simulink model "SF013A_PullCmpActv"  (R2013b)
settings: Solver=FixedStepDiscrete  SolverMode=SingleTasking  StartTime=0.0  StopTime=1  FixedStep=0.002  RelTol=1e-3
values from neighbouring files (symbols this model uses):
  ARCHGLBPRM_100MILLISEC_SEC_F32 = DataDict.Constant    [SF013A_PullCmpActv_DataDict.m]
  ARCHGLBPRM_2MILLISEC_SEC_F32 = DataDict.Constant    [SF013A_PullCmpActv_DataDict.m]
  ARCHGLBPRM_FLOATZEROTHD_ULS_F32 = DataDict.Constant    [SF013A_PullCmpActv_DataDict.m]
  INTGTRSCARSHOTERM_ULS_F32 = DataDict.Constant    [SF013A_PullCmpActv_DataDict.m]
  LONGTERMINTGTRSCAR_ULS_F32 = DataDict.Constant    [SF013A_PullCmpActv_DataDict.m]
  MICROSECTOSEC_ULS_F32 = DataDict.Constant    [SF013A_PullCmpActv_DataDict.m]
  MINSTOSEC_SECPERMINS_F32 = DataDict.Constant    [SF013A_PullCmpActv_DataDict.m]
  PullCmpActvCmpLrnTiDecShoTerm = DataDict.Calibration    [SF013A_PullCmpActv_DataDict.m]
  PullCmpActvCmpLrnTiIncShoTerm = DataDict.Calibration    [SF013A_PullCmpActv_DataDict.m]
  PullCmpActvCmpLrnTiLongTerm = DataDict.Calibration    [SF013A_PullCmpActv_DataDict.m]
  PullCmpActvCmpShoTermRstHwAgThd = DataDict.Calibration    [SF013A_PullCmpActv_DataDict.m]
  PullCmpActvCmpShoTermRstHwTqThd = DataDict.Calibration    [SF013A_PullCmpActv_DataDict.m]
  PullCmpActvCmpShoTermRstLatAThd = DataDict.Calibration    [SF013A_PullCmpActv_DataDict.m]
  PullCmpActvCmpShoTermRstYawRateThd = DataDict.Calibration    [SF013A_PullCmpActv_DataDict.m]
  PullCmpActvEna = DataDict.Calibration    [SF013A_PullCmpActv_DataDict.m]
  PullCmpActvLongTermLim = DataDict.Calibration    [SF013A_PullCmpActv_DataDict.m]
  PullCmpActvLrngEnaAgConfMinMgn = DataDict.Calibration    [SF013A_PullCmpActv_DataDict.m]
  PullCmpActvLrngEnaHwAgMaxMgn = DataDict.Calibration    [SF013A_PullCmpActv_DataDict.m]
  PullCmpActvLrngEnaHwTqMaxMgn = DataDict.Calibration    [SF013A_PullCmpActv_DataDict.m]
  PullCmpActvLrngEnaHwVelMaxMgn = DataDict.Calibration    [SF013A_PullCmpActv_DataDict.m]
  PullCmpActvLrngEnaLatAMaxMgn = DataDict.Calibration    [SF013A_PullCmpActv_DataDict.m]
  PullCmpActvLrngEnaTiThd = DataDict.Calibration    [SF013A_PullCmpActv_DataDict.m]
  PullCmpActvLrngEnaVehSpdMaxMgn = DataDict.Calibration    [SF013A_PullCmpActv_DataDict.m]
  PullCmpActvLrngEnaVehSpdMinMgn = DataDict.Calibration    [SF013A_PullCmpActv_DataDict.m]
  PullCmpActvLrngEnaVehSpdRateMaxMgn = DataDict.Calibration    [SF013A_PullCmpActv_DataDict.m]
  PullCmpActvLrngEnaYawRateMaxMgn = DataDict.Calibration    [SF013A_PullCmpActv_DataDict.m]
  PullCmpActvOpstSignTiShoTerm = DataDict.Calibration    [SF013A_PullCmpActv_DataDict.m]
  PullCmpActvOutpMaxRate = DataDict.Calibration    [SF013A_PullCmpActv_DataDict.m]
  PullCmpActvPullCmpShoTermLim = DataDict.Calibration    [SF013A_PullCmpActv_DataDict.m]
  PullCmpActvPullCmpTotLim = DataDict.Calibration    [SF013A_PullCmpActv_DataDict.m]
  PullCmpActvPullErrLimLongTerm = DataDict.Calibration    [SF013A_PullCmpActv_DataDict.m]
  PullCmpActvPullErrMgnThd = DataDict.Calibration    [SF013A_PullCmpActv_DataDict.m]
  PullCmpActvPullErrShoTermLim = DataDict.Calibration    [SF013A_PullCmpActv_DataDict.m]
  PullCmpActvShoTermRampTi = DataDict.Calibration    [SF013A_PullCmpActv_DataDict.m]
  SysGlbPrmSysTqRat = DataDict.ImprtdCal    [SF013A_PullCmpActv_DataDict.m]
libraries: NxtrAbslt x9, Fil x8, NxtrLim x6, FixdToFloat x3, NxtrSign x3, NxtrMin x3, NxtrNvM x2, NxtrMax x2, simulink x1, FloatToFixd x1, LnrIntrpn x1
(part 1 of 3)
settings Model: Creator=DZVCQL  LastModifiedBy=XZB1DB
settings SolverCC: AutoInsertRateTranBlk=on  InsertRTBMode=Always
settings DataIOCC: LimitDataPoints=off  SaveFormat=Structure  ReturnWorkspaceOutputs=on
settings OptimizationCC: BlockReduction=off  InlineParams=on  ZeroExternalMemoryAtStartup=off  ZeroInternalMemoryAtStartup=off  OptimizeModelRefInitCode=on  LifeSpan=1
settings DebuggingCC: SignalInfNanChecking=error  SignalRangeChecking=warning  ReadBeforeWriteMsg=DisableAll  WriteAfterWriteMsg=DisableAll  WriteAfterReadMsg=DisableAll  UnderspecifiedInitializationDetection=Simplified  SolverPrmCheckMsg=error  InheritedTsInSrcMsg=error  DiscreteInheritContinuousMsg=error  SingleTaskRateTransMsg=error  TasksWithSamePriorityMsg=error  SigSpecEnsureSampleTimeMsg=error  CheckMatrixSingularityMsg=error  ParameterUnderflowMsg=error  ParameterPrecisionLossMsg=error  ParameterTunabilityLossMsg=error  FixptConstUnderflowMsg=warning  FixptConstOverflowMsg=warning  VectorMatrixConversionMsg=error  SignalLabelMismatchMsg=error  UnconnectedInputMsg=error  UnconnectedOutputMsg=error  UnconnectedLineMsg=error  SFcnCompatibilityMsg=error  UniqueDataStoreMsg=warning  BusObjectLabelMismatch=error  RootOutportRequireBusObject=error  AssertControl=DisableAll  ModelReferenceIOMsg=error  ModelReferenceVersionMismatchMessage=warning  ModelReferenceIOMismatchMessage=error  ModelReferenceCSMismatchMessage=warning  ModelReferenceDataLoggingMessage=error  StateNameClashWarn=warning  StrictBusMsg=ErrorOnBusTreatedAsVector  NonBusSignalsTreatedAsBus=error  SFUnexpectedBacktrackingDiag=error  SFInvalidInputDataAccessInChartInitDiag=error  SFNoUnconditionalDefaultTransitionDiag=error  SFTransitionOutsideNaturalParentDiag=error  SFUnconditionalTransitionShadowingDiag=error  SFUndirectedBroadcastEventsDiag=error
settings ModelReferenceCC: ModelReferenceNumInstancesAllowed=Single
settings RTWCC: SystemTargetFile=autosar.tlc  GenCodeOnly=on  TemplateMakefile=ert_default_tmf  Description=AUTOSAR  GenerateReport=on  ProcessScript=autosar_make_rtw_hook  LaunchReport=on
settings CodeAppCC: GenerateComments=off  IgnoreCustomStorageClasses=off  CustomSymbolStrType=$N$R$M  CustomSymbolStrBlkIO=$N$M  SimulinkBlockComments=off
settings STFCustomTargetCC: ParMdlRefBuildCompliant=on  CompOptLevelCompliant=on  IncludeMdlTerminateFcn=off  CombineOutputUpdateFcns=on  SuppressErrorStatus=on  ERTFirstTimeCompliant=on  ERTCustomFileBanners=on  SupportNonFinite=off  SupportComplex=off  SupportContinuousTime=off  SupportNonInlinedSFcns=off  MATLABClassNameForMDSCustomization=Simulink.SoftwareTarget.ERTCustomization  AutosarCompliant=on  GRTInterface=off  SystemTargetFile=autosar.tlc
settings ERTTargetCC: CodeReplacementLibrary=ANSI_C  ConcurrentExecutionCompliant=off  IncludeMdlTerminateFcn=off  SuppressErrorStatus=on  SupportNonFinite=off  SupportComplex=off  ModelStepFunctionPrototypeControlCompliant=off  CPPClassGenCompliant=off  AutosarCompliant=on  InlinedParameterPlacement=NonHierarchical  ERTCustomFileTemplate=example_file_process.tlc  EnableUserReplacementTypes=on

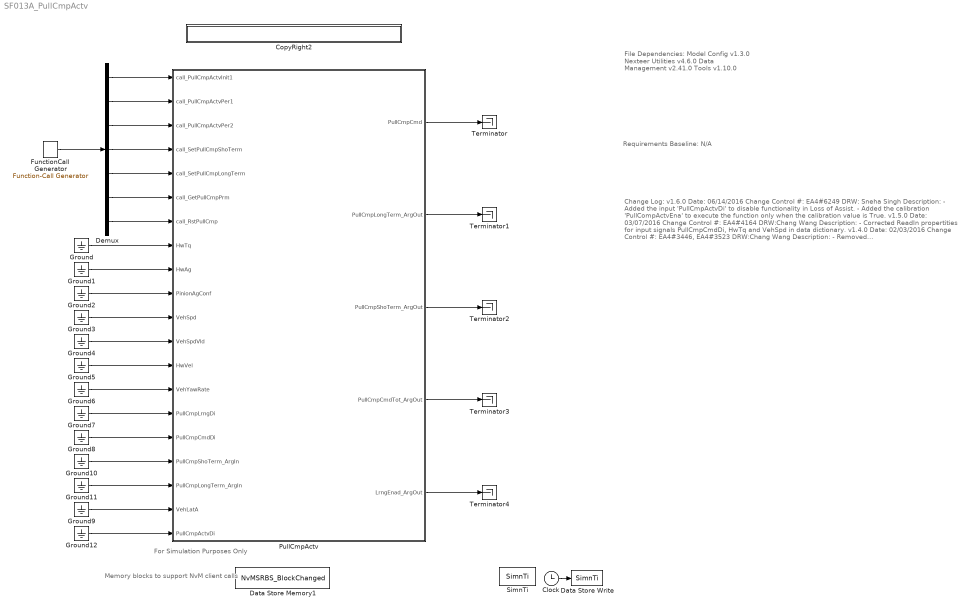
== system SF013A_PullCmpActv ==
  note: Memory blocks to support NvM client calls
  note: For Simulation Purposes Only
  note: File Dependencies:
      |
      | Model Config v1.3.0
      | Nexteer Utilities v4.6.0
      | Data Management v2.41.0
      | Tools v1.10.0
  note: Requirements Baseline: N/A
  note: Change Log:
      |
      | v1.6.0
      | Date: 06/14/2016
      | Change Control #: EA4#6249
      | DRW: Sneha Singh
      | Description:
      | - Added the input 'PullCmpActvDi' to disable functionality in Loss of Assist.
      | - Added the calibration 'PullCompActvEna' to execute the function only when the calibration value is True.
      |
      | v1.5.0
      | Date: 03/07/2016
      | Change Control #: EA4#4164
      | DRW:Chang Wang
      | Description:
      | - Corrected ReadIn propertities for input signals PullCmpCmdDi, HwTq and VehSpd in data dictionary.
      |
      |
      | v1.4.0
      | Date: 02/03/2016
      | Change Control #: EA4#3446, EA4#3523
      | DRW:Chang Wang
      | Description:
      | - Removed PullCmpActvCmpShoTermRstYawRate in the data dictionary as duplicated calibration.
      | - Added VehLatA as the new input to the function for the new functionality, enabling  learning and reset short term learning based on lateral acceleration.
      | - Changed min and max value for PIM PullCmpCmdTot.
      | - Enabled StateMustResolveToSignalObject for IntgtrGainIncShoTerm and IntgtrGainDecShoTerm.
      |
      |
      | v1.3.0
      | Date: 10/15/2015
      | Change Control #: EA4#1967
      | DRW: Price Lefler
      | Description:
      | - Fixed DocUnits for RefTiEnaLrng,  RefTiOpstSign and PullCmpActvOpstSignTiShoTerm.
      | - Fixed design error in the calculation of the short term increasing and decreasing integral gains.
      |
      |
      | v1.2.0
      | Date: 10/2/2015
      | Change Control #: EA4#1009
      | DRW: Price Lefler
      | Description:
      | - Removed GetErrorStatus as a client call in the data dictionary.
      |
      | v1.1.0
      | Date: 9/28/2015
      | Change Control #: EA4#1009
      | DRW: Price Lefler
      | Description:
      | - Timer function usage fixed.
      | - ReadIn and WrittenIn properties fixed for the IRV RampDwnStepSize.
      | - Not equal to comparisons for floating point numbers removed and replaced with a difference and a comparison to ARCHGLBPRM_FLOATZEROTHD_ULS_F32
      | - Removed check of GetErrorStatus for PullCmpLongTerm in the model.
      | - Removed the link to undesired requirement.
      |
      | v1.0.0
      | Date:
      | Change Control #: EA4#1009
      | DRW: Chang Wang
      | Description:
      | - Initial Release
      | - Created from EA3 v003
      | - Level 1 model
  Clock : Clock
  CopyRight2 : Subsystem  Description=|  mask(Copyright Information){none=on}
      | Copyright info block.                                               
      |                                                                     
      | Place copyright information at the top of every subsystem in design.
      mask prompts: none "No parameters"
      mask help: Place copyright information at the top of every subsystem in design.
      mask Display:
      | NxtrConf = 'Nexteer Confidential';
      | 
      | sys = bdroot; %handle for the current model ("system")
      | first = get_param(sys,'Created');
      | if(isempty(first))
      |     first = datestr(now,'yyyy');
      | else
      |     first = first(end-3:end);  %year is last four digits
      | end
      | 
      | last = get_param(sys,'LastModifiedDate');
      | if isempty(last)
      |     last = datestr(now,'yyyy');
      | else
      |     last = last(end-3:end);
      | end
      | 
      | if strcmp(first,last)
      |     fprintf('%s -- Copyright %s Nexteer',NxtrConf,first)
      | else
      |     fprintf('%s -- %s%s- %s Nexteer',NxtrConf,char(169),first,last)
      | end
  Data Store Memory1 : DataStoreMemory  DataStoreName=NvMSRBS_BlockChanged  ReadBeforeWriteMsg=warning  WriteAfterWriteMsg=warning  WriteAfterReadMsg=warning
  Data Store Write : DataStoreWrite  DataStoreName=SimnTi
  Demux : Demux  Outputs=7
  FunctionCall Generator : simulink/Ports & Subsystems/Function-Call Generator  sample_time=0.002  numberOfIterations=1
  Ground{,1..12} (13 alike) : Ground
  PullCmpActv : Subsystem
  SimnTi : DataStoreMemory  DataStoreName=SimnTi
  Terminator{,1..4} (5 alike) : Terminator
  wires:
  Clock/1 -> Data Store Write/1
  Demux/1 -> PullCmpActv/1(call_PullCmpActvInit1)
  Demux/2 -> PullCmpActv/2(call_PullCmpActvPer1)
  FunctionCall Generator/1 -> Demux/1
  Demux/3 -> PullCmpActv/3(call_PullCmpActvPer2)
  Demux/4 -> PullCmpActv/4(call_SetPullCmpShoTerm)
  Demux/5 -> PullCmpActv/5(call_SetPullCmpLongTerm)
  Demux/6 -> PullCmpActv/6(call_GetPullCmpPrm)
  Ground/1 -> PullCmpActv/8(HwTq)
  Ground1/1 -> PullCmpActv/9(HwAg)
  Ground2/1 -> PullCmpActv/10(PinionAgConf)
  Ground3/1 -> PullCmpActv/11(VehSpd)
  Ground4/1 -> PullCmpActv/12(VehSpdVld)
  Ground5/1 -> PullCmpActv/13(HwVel)
  Ground6/1 -> PullCmpActv/14(VehYawRate)
  Ground7/1 -> PullCmpActv/15(PullCmpLrngDi)
  Ground8/1 -> PullCmpActv/16(PullCmpCmdDi)
  Ground10/1 -> PullCmpActv/17(PullCmpShoTerm_ArgIn)
  Ground11/1 -> PullCmpActv/18(PullCmpLongTerm_ArgIn)
  PullCmpActv/1(PullCmpCmd) -> Terminator/1
  PullCmpActv/2(PullCmpLongTerm_ArgOut) -> Terminator1/1
  PullCmpActv/3(PullCmpShoTerm_ArgOut) -> Terminator2/1
  PullCmpActv/4(PullCmpCmdTot_ArgOut) -> Terminator3/1
  PullCmpActv/5(LrngEnad_ArgOut) -> Terminator4/1
  Demux/7 -> PullCmpActv/7(call_RstPullCmp)
  Ground9/1 -> PullCmpActv/19(VehLatA)
  Ground12/1 -> PullCmpActv/20(PullCmpActvDi)

== system SF013A_PullCmpActv/CopyRight2 ==

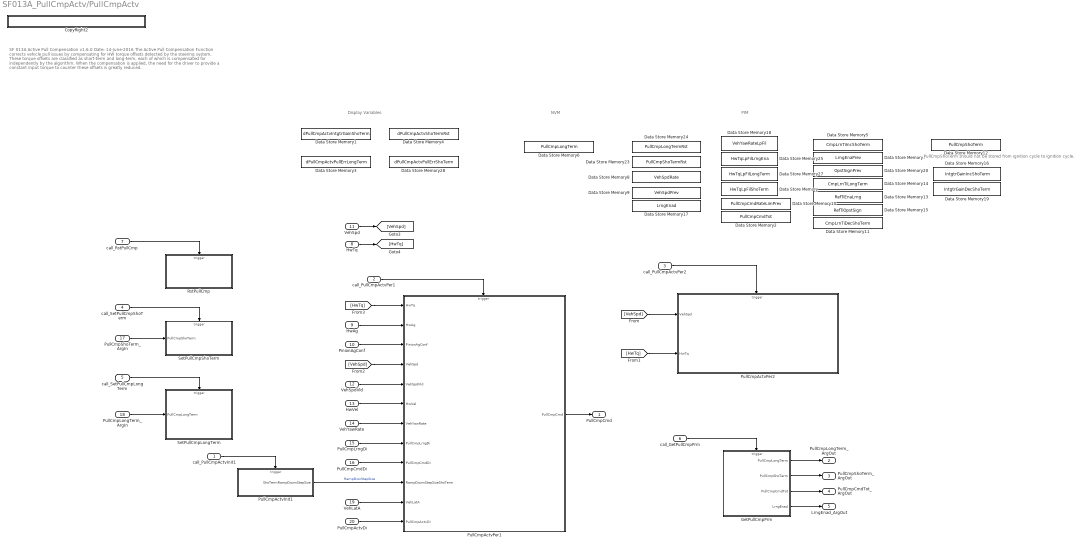
== system SF013A_PullCmpActv/PullCmpActv ==
  note: PullCmpShoTerm should not be stored from ignition cycle to ignition cycle.
  note: Display Variables
  note: SF 013A  Active Pull Compensation
      | v1.6.0      Date: 14-June-2016
      |
      | The Active Pull Compensation Function corrects vehicle pull issues by compensating for HW torque offsets detected by the steering system.
      | These torque offsets are classified as short-term and long-term, each of which is compensated for independently by the algorithm.  When
      | the compensation is applied, the need for the driver to provide a constant input torque to counter these offsets is greatly reduced.
  note: NVM
  note: PIM
  call_PullCmpActvInit1 : Inport
  call_PullCmpActvPer1 : Inport  Port=2
  call_PullCmpActvPer2 : Inport  Port=3
  call_SetPullCmpShoTerm : Inport  Port=4
  call_SetPullCmpLongTerm : Inport  Port=5
  call_GetPullCmpPrm : Inport  Port=6
  call_RstPullCmp : Inport  Port=7
  HwTq : Inport  Port=8
  HwAg : Inport  Port=9
  PinionAgConf : Inport  Port=10
  VehSpd : Inport  Port=11
  VehSpdVld : Inport  Port=12
  HwVel : Inport  Port=13
  VehYawRate : Inport  Port=14
  PullCmpLrngDi : Inport  Port=15
  PullCmpCmdDi : Inport  Port=16
  PullCmpShoTerm_ArgIn : Inport  Port=17
  PullCmpLongTerm_ArgIn : Inport  Port=18
  VehLatA : Inport  Port=19
  PullCmpActvDi : Inport  Port=20
  CopyRight2 : Subsystem  Description=|  mask(Copyright Information){none=on}
      | Copyright info block.                                               
      |                                                                     
      | Place copyright information at the top of every subsystem in design.
      mask prompts: none "No parameters"
      mask help: Place copyright information at the top of every subsystem in design.
      mask Display:
      | NxtrConf = 'Nexteer Confidential';
      | 
      | sys = bdroot; %handle for the current model ("system")
      | first = get_param(sys,'Created');
      | if(isempty(first))
      |     first = datestr(now,'yyyy');
      | else
      |     first = first(end-3:end);  %year is last four digits
      | end
      | 
      | last = get_param(sys,'LastModifiedDate');
      | if isempty(last)
      |     last = datestr(now,'yyyy');
      | else
      |     last = last(end-3:end);
      | end
      | 
      | if strcmp(first,last)
      |     fprintf('%s -- Copyright %s Nexteer',NxtrConf,first)
      | else
      |     fprintf('%s -- %s%s- %s Nexteer',NxtrConf,char(169),first,last)
      | end
  Data Store Memory : DataStoreMemory  DataStoreName=HwTqLpFilShoTerm  ReadBeforeWriteMsg=warning  WriteAfterWriteMsg=warning  WriteAfterReadMsg=warning  InitialValue=[]  StateMustResolveToSignalObject=on
  Data Store Memory1 : DataStoreMemory  DataStoreName=dPullCmpActvIntgtrGainShoTerm  ReadBeforeWriteMsg=warning  WriteAfterWriteMsg=warning  WriteAfterReadMsg=warning  StateMustResolveToSignalObject=on
  Data Store Memory10 : DataStoreMemory  DataStoreName=PullCmpCmdRateLimPrev  ReadBeforeWriteMsg=warning  WriteAfterWriteMsg=warning  WriteAfterReadMsg=warning  StateMustResolveToSignalObject=on
  Data Store Memory11 : DataStoreMemory  DataStoreName=CmpLrnTiDecShoTerm  ReadBeforeWriteMsg=warning  WriteAfterWriteMsg=warning  WriteAfterReadMsg=warning  StateMustResolveToSignalObject=on
  Data Store Memory12 : DataStoreMemory  DataStoreName=PullCmpShoTerm  ReadBeforeWriteMsg=warning  WriteAfterWriteMsg=warning  WriteAfterReadMsg=warning  StateMustResolveToSignalObject=on
  Data Store Memory13 : DataStoreMemory  DataStoreName=RefTiEnaLrng  ReadBeforeWriteMsg=warning  WriteAfterWriteMsg=warning  WriteAfterReadMsg=warning  StateMustResolveToSignalObject=on
  Data Store Memory14 : DataStoreMemory  DataStoreName=CmpLrnTiLongTerm  ReadBeforeWriteMsg=warning  WriteAfterWriteMsg=warning  WriteAfterReadMsg=warning  StateMustResolveToSignalObject=on
  Data Store Memory15 : DataStoreMemory  DataStoreName=RefTiOpstSign  ReadBeforeWriteMsg=warning  WriteAfterWriteMsg=warning  WriteAfterReadMsg=warning  StateMustResolveToSignalObject=on
  Data Store Memory16 : DataStoreMemory  DataStoreName=IntgtrGainIncShoTerm  ReadBeforeWriteMsg=warning  WriteAfterWriteMsg=warning  WriteAfterReadMsg=warning  StateMustResolveToSignalObject=on
  Data Store Memory17 : DataStoreMemory  DataStoreName=LrngEnad  ReadBeforeWriteMsg=warning  WriteAfterWriteMsg=warning  WriteAfterReadMsg=warning  StateMustResolveToSignalObject=on
  Data Store Memory18 : DataStoreMemory  DataStoreName=VehYawRateLpFil  ReadBeforeWriteMsg=warning  WriteAfterWriteMsg=warning  WriteAfterReadMsg=warning  InitialValue=[]  StateMustResolveToSignalObject=on
  Data Store Memory19 : DataStoreMemory  DataStoreName=IntgtrGainDecShoTerm  ReadBeforeWriteMsg=warning  WriteAfterWriteMsg=warning  WriteAfterReadMsg=warning  StateMustResolveToSignalObject=on
  Data Store Memory2 : DataStoreMemory  DataStoreName=PullCmpCmdTot  ReadBeforeWriteMsg=warning  WriteAfterWriteMsg=warning  WriteAfterReadMsg=warning  StateMustResolveToSignalObject=on
  Data Store Memory20 : DataStoreMemory  DataStoreName=OpstSignPrev  ReadBeforeWriteMsg=warning  WriteAfterWriteMsg=warning  WriteAfterReadMsg=warning  StateMustResolveToSignalObject=on
  Data Store Memory23 : DataStoreMemory  DataStoreName=PullCmpShoTermRst  ReadBeforeWriteMsg=warning  WriteAfterWriteMsg=warning  WriteAfterReadMsg=warning  StateMustResolveToSignalObject=on
  Data Store Memory24 : DataStoreMemory  DataStoreName=PullCmpLongTermRst  ReadBeforeWriteMsg=warning  WriteAfterWriteMsg=warning  WriteAfterReadMsg=warning  StateMustResolveToSignalObject=on
  Data Store Memory25 : DataStoreMemory  DataStoreName=HwTqLpFilLrngEna  ReadBeforeWriteMsg=warning  WriteAfterWriteMsg=warning  WriteAfterReadMsg=warning  InitialValue=[]  StateMustResolveToSignalObject=on
  Data Store Memory27 : DataStoreMemory  DataStoreName=HwTqLpFilLongTerm  ReadBeforeWriteMsg=warning  WriteAfterWriteMsg=warning  WriteAfterReadMsg=warning  InitialValue=[]  StateMustResolveToSignalObject=on
  Data Store Memory28 : DataStoreMemory  DataStoreName=dPullCmpActvPullErrShoTerm  ReadBeforeWriteMsg=warning  WriteAfterWriteMsg=warning  WriteAfterReadMsg=warning  StateMustResolveToSignalObject=on
  Data Store Memory3 : DataStoreMemory  DataStoreName=dPullCmpActvPullErrLongTerm  ReadBeforeWriteMsg=warning  WriteAfterWriteMsg=warning  WriteAfterReadMsg=warning  StateMustResolveToSignalObject=on
  Data Store Memory4 : DataStoreMemory  DataStoreName=dPullCmpActvShoTermRst  ReadBeforeWriteMsg=warning  WriteAfterWriteMsg=warning  WriteAfterReadMsg=warning  StateMustResolveToSignalObject=on
  Data Store Memory5 : DataStoreMemory  DataStoreName=CmpLrnTiIncShoTerm  ReadBeforeWriteMsg=warning  WriteAfterWriteMsg=warning  WriteAfterReadMsg=warning  StateMustResolveToSignalObject=on
  Data Store Memory6 : DataStoreMemory  DataStoreName=PullCmpLongTerm  ReadBeforeWriteMsg=warning  WriteAfterWriteMsg=warning  WriteAfterReadMsg=warning  StateMustResolveToSignalObject=on
  Data Store Memory7 : DataStoreMemory  DataStoreName=LrngEnaPrev  ReadBeforeWriteMsg=warning  WriteAfterWriteMsg=warning  WriteAfterReadMsg=warning  StateMustResolveToSignalObject=on
  Data Store Memory8 : DataStoreMemory  DataStoreName=VehSpdRate  ReadBeforeWriteMsg=warning  WriteAfterWriteMsg=warning  WriteAfterReadMsg=warning  StateMustResolveToSignalObject=on
  Data Store Memory9 : DataStoreMemory  DataStoreName=VehSpdPrev  ReadBeforeWriteMsg=warning  WriteAfterWriteMsg=warning  WriteAfterReadMsg=warning  StateMustResolveToSignalObject=on
  GetPullCmpPrm : Subsystem  TreatAsAtomicUnit=on
  PullCmpActvInit1 : Subsystem  TreatAsAtomicUnit=on
  PullCmpActvPer1 : Subsystem  TreatAsAtomicUnit=on
  PullCmpActvPer2 : Subsystem  TreatAsAtomicUnit=on
  RstPullCmp : Subsystem  TreatAsAtomicUnit=on
  SetPullCmpLongTerm : Subsystem  TreatAsAtomicUnit=on
  SetPullCmpShoTerm : Subsystem  TreatAsAtomicUnit=on
  PullCmpCmd : Outport
  PullCmpLongTerm_ArgOut : Outport  Port=2
  PullCmpShoTerm_ArgOut : Outport  Port=3
  PullCmpCmdTot_ArgOut : Outport  Port=4
  LrngEnad_ArgOut : Outport  Port=5
  wires:
  GetPullCmpPrm/4(LrngEnad) -> LrngEnad_ArgOut/1
  GetPullCmpPrm/3(PullCmpCmdTot) -> PullCmpCmdTot_ArgOut/1
  GetPullCmpPrm/2(PullCmpShoTerm) -> PullCmpShoTerm_ArgOut/1
  GetPullCmpPrm/1(PullCmpLongTerm) -> PullCmpLongTerm_ArgOut/1
  call_PullCmpActvPer1/1 -> PullCmpActvPer1/Trigger
  call_PullCmpActvInit1/1 -> PullCmpActvInit1/Trigger
  call_PullCmpActvPer2/1 -> PullCmpActvPer2/Trigger
  call_SetPullCmpShoTerm/1 -> SetPullCmpShoTerm/Trigger
  call_SetPullCmpLongTerm/1 -> SetPullCmpLongTerm/Trigger
  call_GetPullCmpPrm/1 -> GetPullCmpPrm/Trigger
  HwTq/1 -> [HwTq]
  HwAg/1 -> PullCmpActvPer1/2("HwAg ")
  PinionAgConf/1 -> PullCmpActvPer1/3("PinionAgConf ")
  VehSpd/1 -> [VehSpd]
  VehSpdVld/1 -> PullCmpActvPer1/5(VehSpdVld)
  HwVel/1 -> PullCmpActvPer1/6(HwVel)
  VehYawRate/1 -> PullCmpActvPer1/7(VehYawRate)
  PullCmpLrngDi/1 -> PullCmpActvPer1/8(PullCmpLrngDi)
  [VehSpd] -> PullCmpActvPer2/1(VehSpd)
  [HwTq] -> PullCmpActvPer2/2(HwTq)
  PullCmpShoTerm_ArgIn/1 -> SetPullCmpShoTerm/1(PullCmpShoTerm)
  PullCmpLongTerm_ArgIn/1 -> SetPullCmpLongTerm/1(PullCmpLongTerm)
  call_RstPullCmp/1 -> RstPullCmp/Trigger
  PullCmpActvPer1/1(PullCmpCmd) -> PullCmpCmd/1
  PullCmpCmdDi/1 -> PullCmpActvPer1/9(PullCmpCmdDi)
  [VehSpd] -> PullCmpActvPer1/4(VehSpd)
  [HwTq] -> PullCmpActvPer1/1(HwTq)
  PullCmpActvInit1/1(ShoTermRampDownStepSize) -> PullCmpActvPer1/10(RampDownStepSizeShoTerm)  "RampDwnStepSize"
  VehLatA/1 -> PullCmpActvPer1/11(VehLatA)
  PullCmpActvDi/1 -> PullCmpActvPer1/12(PullCmpActvDi)

== system SF013A_PullCmpActv/PullCmpActv/CopyRight2 ==

== system SF013A_PullCmpActv/PullCmpActv/GetPullCmpPrm ==
  function : TriggerPort  TriggerType=function-call
  CopyRight2 : Subsystem  Description=|  mask(Copyright Information){none=on}
      | Copyright info block.                                               
      |                                                                     
      | Place copyright information at the top of every subsystem in design.
      mask prompts: none "No parameters"
      mask help: Place copyright information at the top of every subsystem in design.
      mask Display:
      | NxtrConf = 'Nexteer Confidential';
      | 
      | sys = bdroot; %handle for the current model ("system")
      | first = get_param(sys,'Created');
      | if(isempty(first))
      |     first = datestr(now,'yyyy');
      | else
      |     first = first(end-3:end);  %year is last four digits
      | end
      | 
      | last = get_param(sys,'LastModifiedDate');
      | if isempty(last)
      |     last = datestr(now,'yyyy');
      | else
      |     last = last(end-3:end);
      | end
      | 
      | if strcmp(first,last)
      |     fprintf('%s -- Copyright %s Nexteer',NxtrConf,first)
      | else
      |     fprintf('%s -- %s%s- %s Nexteer',NxtrConf,char(169),first,last)
      | end
  Data Store Read : DataStoreRead  DataStoreName=PullCmpLongTerm
  Data Store Read1 : DataStoreRead  DataStoreName=PullCmpShoTerm
  Data Store Read2 : DataStoreRead  DataStoreName=PullCmpCmdTot
  Data Store Read3 : DataStoreRead  DataStoreName=LrngEnad
  PullCmpLongTerm : Outport
  PullCmpShoTerm : Outport  Port=2
  PullCmpCmdTot : Outport  Port=3
  LrngEnad : Outport  Port=4
  wires:
  Data Store Read/1 -> PullCmpLongTerm/1
  Data Store Read3/1 -> LrngEnad/1
  Data Store Read2/1 -> PullCmpCmdTot/1
  Data Store Read1/1 -> PullCmpShoTerm/1

== system SF013A_PullCmpActv/PullCmpActv/PullCmpActvInit1 ==
  note: Call to GetErrorStatus removed because error handling for NvM block should be taken care of
      | by the NvM Manager as per the Data Dictionary.
  function : TriggerPort  TriggerType=function-call
  Constant1 : Constant  Value=PullCmpActvPullCmpShoTermLim
  Constant3 : Constant  Value=PullCmpActvShoTermRampTi
  Constant4 : Constant  Value=ARCHGLBPRM_2MILLISEC_SEC_F32
  Constant5 : Constant  RequirementInfo={} %GIDa_7dd5e1a6_3745_4149_8da9_62934d4976cf  OutDataTypeStr=single
  CopyRight2 : Subsystem  Description=|  mask(Copyright Information){none=on}
      | Copyright info block.                                               
      |                                                                     
      | Place copyright information at the top of every subsystem in design.
      mask prompts: none "No parameters"
      mask help: Place copyright information at the top of every subsystem in design.
      mask Display:
      | NxtrConf = 'Nexteer Confidential';
      | 
      | sys = bdroot; %handle for the current model ("system")
      | first = get_param(sys,'Created');
      | if(isempty(first))
      |     first = datestr(now,'yyyy');
      | else
      |     first = first(end-3:end);  %year is last four digits
      | end
      | 
      | last = get_param(sys,'LastModifiedDate');
      | if isempty(last)
      |     last = datestr(now,'yyyy');
      | else
      |     last = last(end-3:end);
      | end
      | 
      | if strcmp(first,last)
      |     fprintf('%s -- Copyright %s Nexteer',NxtrConf,first)
      | else
      |     fprintf('%s -- %s%s- %s Nexteer',NxtrConf,char(169),first,last)
      | end
  Divide1 : Product  Inputs=**/
  PullCmpActvHwTqFilLpInit : Fil/FilLpInit  Ic=0  Ts=ARCHGLBPRM_2MILLISEC_SEC_F32  Freq=PullCmpActvHwTqFilFrqLrngEna  StVar=HwTqLpFilLrngEna
  PullCmpActvHwTqLongTermFilLpInit : Fil/FilLpInit  Ic=0  Ts=ARCHGLBPRM_100MILLISEC_SEC_F32  Freq=PullCmpActvHwTqFilFrqLongTerm  StVar=HwTqLpFilLongTerm
  PullCmpActvHwTqShoTermFilLpInit : Fil/FilLpInit  Ic=0  Ts=ARCHGLBPRM_2MILLISEC_SEC_F32  Freq=PullCmpActvHwTqFilFrqShoTerm  StVar=HwTqLpFilShoTerm
  PullCmpActvYawRateFilLpInit : Fil/FilLpInit  Ic=0  Ts=ARCHGLBPRM_2MILLISEC_SEC_F32  Freq=PullCmpActvYawRateFilFrq  StVar=VehYawRateLpFil
  PullCmpLongTerm_SetRamBlockStatus : NxtrNvM/Set Ram Block Status  RequirementInfo={} %GIDa_d378c946_11fa_4093_99df_efb6ba3e3b6f  FuncName=Set Ram Block Status  NvMBlockName=PullCmpLongTerm  VoidFuncRtn=on  BlockChanged_DSN=NvMSRBS_BlockChanged  Return_DSN=NvMSRBS_Return
      settings: AttributesFormatString=%<FuncName>
  ShoTermRampDownStepSize : Outport
  wires:
  Constant4/1 -> Divide1/1
  Constant3/1 -> Divide1/3
  Constant1/1 -> Divide1/2
  Divide1/1 -> ShoTermRampDownStepSize/1
  Constant5/1 -> PullCmpLongTerm_SetRamBlockStatus/1

== system SF013A_PullCmpActv/PullCmpActv/PullCmpActvPer1 ==
  HwTq : Inport
  "HwAg " : Inport  Port=2
  "PinionAgConf " : Inport  Port=3
  VehSpd : Inport  Port=4
  VehSpdVld : Inport  Port=5
  HwVel : Inport  Port=6
  VehYawRate : Inport  Port=7
  PullCmpLrngDi : Inport  Port=8
  PullCmpCmdDi : Inport  Port=9
  RampDownStepSizeShoTerm : Inport  Port=10
  VehLatA : Inport  Port=11
  PullCmpActvDi : Inport  Port=12
  function : TriggerPort  TriggerType=function-call
  Constant3 : Constant  Value=PullCmpActvEna
  CopyRight2 : Subsystem  Description=|  mask(Copyright Information){none=on}
      | Copyright info block.                                               
      |                                                                     
      | Place copyright information at the top of every subsystem in design.
      mask prompts: none "No parameters"
      mask help: Place copyright information at the top of every subsystem in design.
      mask Display:
      | NxtrConf = 'Nexteer Confidential';
      | 
      | sys = bdroot; %handle for the current model ("system")
      | first = get_param(sys,'Created');
      | if(isempty(first))
      |     first = datestr(now,'yyyy');
      | else
      |     first = first(end-3:end);  %year is last four digits
      | end
      | 
      | last = get_param(sys,'LastModifiedDate');
      | if isempty(last)
      |     last = datestr(now,'yyyy');
      | else
      |     last = last(end-3:end);
      | end
      | 
      | if strcmp(first,last)
      |     fprintf('%s -- Copyright %s Nexteer',NxtrConf,first)
      | else
      |     fprintf('%s -- %s%s- %s Nexteer',NxtrConf,char(169),first,last)
      | end
  If : If  IfExpression=u1  ShowElse=off
  PullCmpActvPer1 : Subsystem
  PullCmpCmd : Outport
  wires:
  HwTq/1 -> PullCmpActvPer1/1(HwTq)
  "HwAg "/1 -> PullCmpActvPer1/2("HwAg ")
  "PinionAgConf "/1 -> PullCmpActvPer1/3("PinionAgConf ")
  VehSpd/1 -> PullCmpActvPer1/4(VehSpd)
  VehSpdVld/1 -> PullCmpActvPer1/5(VehSpdVld)
  HwVel/1 -> PullCmpActvPer1/6(HwVel)
  VehYawRate/1 -> PullCmpActvPer1/7(VehYawRate)
  PullCmpLrngDi/1 -> PullCmpActvPer1/8(PullCmpLrngDi)
  PullCmpCmdDi/1 -> PullCmpActvPer1/9(PullCmpCmdDi)
  RampDownStepSizeShoTerm/1 -> PullCmpActvPer1/10(RampDownStepSizeShoTerm)
  VehLatA/1 -> PullCmpActvPer1/11(VehLatA)
  PullCmpActvDi/1 -> PullCmpActvPer1/12(PullCmpActvDi)
  PullCmpActvPer1/1(PullCmpCmd) -> PullCmpCmd/1
  If/1 -> PullCmpActvPer1/Action
  Constant3/1 -> If/1

== system SF013A_PullCmpActv/PullCmpActv/PullCmpActvPer2 ==
  VehSpd : Inport
  HwTq : Inport  Port=2
  function : TriggerPort  TriggerType=function-call
  Constant3 : Constant  Value=PullCmpActvEna
  CopyRight2 : Subsystem  Description=|  mask(Copyright Information){none=on}
      | Copyright info block.                                               
      |                                                                     
      | Place copyright information at the top of every subsystem in design.
      mask prompts: none "No parameters"
      mask help: Place copyright information at the top of every subsystem in design.
      mask Display:
      | NxtrConf = 'Nexteer Confidential';
      | 
      | sys = bdroot; %handle for the current model ("system")
      | first = get_param(sys,'Created');
      | if(isempty(first))
      |     first = datestr(now,'yyyy');
      | else
      |     first = first(end-3:end);  %year is last four digits
      | end
      | 
      | last = get_param(sys,'LastModifiedDate');
      | if isempty(last)
      |     last = datestr(now,'yyyy');
      | else
      |     last = last(end-3:end);
      | end
      | 
      | if strcmp(first,last)
      |     fprintf('%s -- Copyright %s Nexteer',NxtrConf,first)
      | else
      |     fprintf('%s -- %s%s- %s Nexteer',NxtrConf,char(169),first,last)
      | end
  If1 : If  IfExpression=u1  ShowElse=off
  PullCmpActvPer2 : Subsystem
  wires:
  If1/1 -> PullCmpActvPer2/Action
  Constant3/1 -> If1/1
  VehSpd/1 -> PullCmpActvPer2/1(VehSpd)
  HwTq/1 -> PullCmpActvPer2/2(HwTq)

== system SF013A_PullCmpActv/PullCmpActv/RstPullCmp ==
  function : TriggerPort  TriggerType=function-call
  Constant : Constant  OutDataTypeStr=boolean
  Constant1 : Constant  OutDataTypeStr=boolean
  CopyRight2 : Subsystem  Description=|  mask(Copyright Information){none=on}
      | Copyright info block.                                               
      |                                                                     
      | Place copyright information at the top of every subsystem in design.
      mask prompts: none "No parameters"
      mask help: Place copyright information at the top of every subsystem in design.
      mask Display:
      | NxtrConf = 'Nexteer Confidential';
      | 
      | sys = bdroot; %handle for the current model ("system")
      | first = get_param(sys,'Created');
      | if(isempty(first))
      |     first = datestr(now,'yyyy');
      | else
      |     first = first(end-3:end);  %year is last four digits
      | end
      | 
      | last = get_param(sys,'LastModifiedDate');
      | if isempty(last)
      |     last = datestr(now,'yyyy');
      | else
      |     last = last(end-3:end);
      | end
      | 
      | if strcmp(first,last)
      |     fprintf('%s -- Copyright %s Nexteer',NxtrConf,first)
      | else
      |     fprintf('%s -- %s%s- %s Nexteer',NxtrConf,char(169),first,last)
      | end
  Data Store Write : DataStoreWrite  DataStoreName=PullCmpShoTermRst
  Data Store Write1 : DataStoreWrite  DataStoreName=PullCmpLongTermRst
  wires:
  Constant1/1 -> Data Store Write1/1
  Constant/1 -> Data Store Write/1

== system SF013A_PullCmpActv/PullCmpActv/SetPullCmpLongTerm ==
  PullCmpLongTerm : Inport
  function : TriggerPort  TriggerType=function-call
  Constant : Constant  RequirementInfo={} %GIDa_9c81615b_60a0_4dde_9f7a_e3ec35a8c376  OutDataTypeStr=single
  CopyRight2 : Subsystem  Description=|  mask(Copyright Information){none=on}
      | Copyright info block.                                               
      |                                                                     
      | Place copyright information at the top of every subsystem in design.
      mask prompts: none "No parameters"
      mask help: Place copyright information at the top of every subsystem in design.
      mask Display:
      | NxtrConf = 'Nexteer Confidential';
      | 
      | sys = bdroot; %handle for the current model ("system")
      | first = get_param(sys,'Created');
      | if(isempty(first))
      |     first = datestr(now,'yyyy');
      | else
      |     first = first(end-3:end);  %year is last four digits
      | end
      | 
      | last = get_param(sys,'LastModifiedDate');
      | if isempty(last)
      |     last = datestr(now,'yyyy');
      | else
      |     last = last(end-3:end);
      | end
      | 
      | if strcmp(first,last)
      |     fprintf('%s -- Copyright %s Nexteer',NxtrConf,first)
      | else
      |     fprintf('%s -- %s%s- %s Nexteer',NxtrConf,char(169),first,last)
      | end
  Data Store Write : DataStoreWrite  DataStoreName=PullCmpLongTerm
  PullCmpLongTerm_SetRamBlockStatus : NxtrNvM/Set Ram Block Status  RequirementInfo={} %GIDa_05a0e1f5_a949_4242_b915_dab1753a43ae  FuncName=Set Ram Block Status  NvMBlockName=PullCmpLongTerm  VoidFuncRtn=on  BlockChanged_DSN=NvMSRBS_BlockChanged  Return_DSN=NvMSRBS_Return
      settings: AttributesFormatString=%<FuncName>
  wires:
  PullCmpLongTerm/1 -> Data Store Write/1
  Constant/1 -> PullCmpLongTerm_SetRamBlockStatus/1

== system SF013A_PullCmpActv/PullCmpActv/SetPullCmpShoTerm ==
  PullCmpShoTerm : Inport
  function : TriggerPort  TriggerType=function-call
  CopyRight2 : Subsystem  Description=|  mask(Copyright Information){none=on}
      | Copyright info block.                                               
      |                                                                     
      | Place copyright information at the top of every subsystem in design.
      mask prompts: none "No parameters"
      mask help: Place copyright information at the top of every subsystem in design.
      mask Display:
      | NxtrConf = 'Nexteer Confidential';
      | 
      | sys = bdroot; %handle for the current model ("system")
      | first = get_param(sys,'Created');
      | if(isempty(first))
      |     first = datestr(now,'yyyy');
      | else
      |     first = first(end-3:end);  %year is last four digits
      | end
      | 
      | last = get_param(sys,'LastModifiedDate');
      | if isempty(last)
      |     last = datestr(now,'yyyy');
      | else
      |     last = last(end-3:end);
      | end
      | 
      | if strcmp(first,last)
      |     fprintf('%s -- Copyright %s Nexteer',NxtrConf,first)
      | else
      |     fprintf('%s -- %s%s- %s Nexteer',NxtrConf,char(169),first,last)
      | end
  Data Store Write : DataStoreWrite  DataStoreName=PullCmpShoTerm
  wires:
  PullCmpShoTerm/1 -> Data Store Write/1

== system SF013A_PullCmpActv/PullCmpActv/GetPullCmpPrm/CopyRight2 ==

== system SF013A_PullCmpActv/PullCmpActv/PullCmpActvInit1/CopyRight2 ==

== system SF013A_PullCmpActv/PullCmpActv/PullCmpActvPer1/CopyRight2 ==

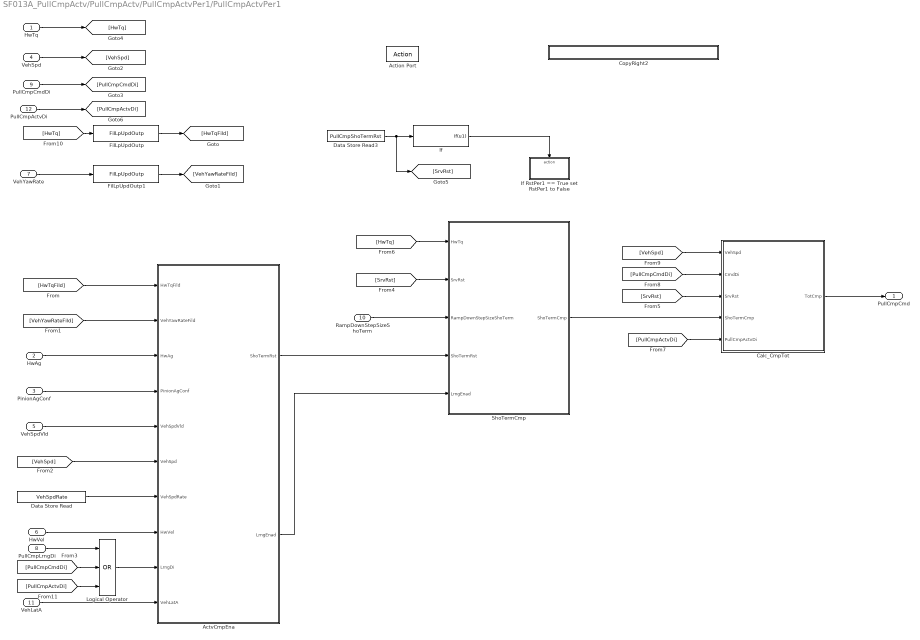
== system SF013A_PullCmpActv/PullCmpActv/PullCmpActvPer1/PullCmpActvPer1 ==
  HwTq : Inport
  "HwAg " : Inport  Port=2
  "PinionAgConf " : Inport  Port=3
  VehSpd : Inport  Port=4
  VehSpdVld : Inport  Port=5
  HwVel : Inport  Port=6
  VehYawRate : Inport  Port=7
  PullCmpLrngDi : Inport  Port=8
  PullCmpCmdDi : Inport  Port=9
  RampDownStepSizeShoTerm : Inport  Port=10
  VehLatA : Inport  Port=11
  PullCmpActvDi : Inport  Port=12
  Action Port : ActionPort  ActionType=then
  ActvCmpEna : Subsystem  TreatAsAtomicUnit=on
  Calc_CmpTot : Subsystem  TreatAsAtomicUnit=on
  CopyRight2 : Subsystem  Description=|  mask(Copyright Information){none=on}
      | Copyright info block.                                               
      |                                                                     
      | Place copyright information at the top of every subsystem in design.
      mask prompts: none "No parameters"
      mask help: Place copyright information at the top of every subsystem in design.
      mask Display:
      | NxtrConf = 'Nexteer Confidential';
      | 
      | sys = bdroot; %handle for the current model ("system")
      | first = get_param(sys,'Created');
      | if(isempty(first))
      |     first = datestr(now,'yyyy');
      | else
      |     first = first(end-3:end);  %year is last four digits
      | end
      | 
      | last = get_param(sys,'LastModifiedDate');
      | if isempty(last)
      |     last = datestr(now,'yyyy');
      | else
      |     last = last(end-3:end);
      | end
      | 
      | if strcmp(first,last)
      |     fprintf('%s -- Copyright %s Nexteer',NxtrConf,first)
      | else
      |     fprintf('%s -- %s%s- %s Nexteer',NxtrConf,char(169),first,last)
      | end
  Data Store Read : DataStoreRead  DataStoreName=VehSpdRate
  Data Store Read3 : DataStoreRead  DataStoreName=PullCmpShoTermRst
  FilLpUpdOutp : Fil/FilLpUpdOutp  StVar=HwTqLpFilLrngEna
      settings: AttributesFormatString=StVar: %<StVar>
  FilLpUpdOutp1 : Fil/FilLpUpdOutp  StVar=VehYawRateLpFil
      settings: AttributesFormatString=StVar: %<StVar>
  If : If  IfExpression=u1  ShowElse=off
  If RstPer1 == True set RstPer1 to False : Subsystem  TreatAsAtomicUnit=on
  Logical Operator : Logic  Operator=OR  Inputs=3  AllPortsSameDT=off  OutDataTypeStr=boolean
  ShoTermCmp : Subsystem  TreatAsAtomicUnit=on
  PullCmpCmd : Outport
  wires:
  HwTq/1 -> [HwTq]
  VehYawRate/1 -> FilLpUpdOutp1/1
  FilLpUpdOutp/1 -> [HwTqFild]
  FilLpUpdOutp1/1 -> [VehYawRateFild]
  [HwTqFild] -> ActvCmpEna/1(HwTqFild)
  [VehYawRateFild] -> ActvCmpEna/2(VehYawRateFild)
  "HwAg "/1 -> ActvCmpEna/3(HwAg)
  "PinionAgConf "/1 -> ActvCmpEna/4(PinionAgConf)
  VehSpdVld/1 -> ActvCmpEna/5(VehSpdVld)
  HwVel/1 -> ActvCmpEna/8(HwVel)
  VehSpd/1 -> [VehSpd]
  [VehSpd] -> ActvCmpEna/6(VehSpd)
  Data Store Read/1 -> ActvCmpEna/7(VehSpdRate)
  PullCmpCmdDi/1 -> [PullCmpCmdDi]
  PullCmpLrngDi/1 -> Logical Operator/1
  Logical Operator/1 -> ActvCmpEna/9(LrngDi)
  [PullCmpCmdDi] -> Logical Operator/2
  [SrvRst] -> ShoTermCmp/2(SrvRst)
  [HwTq] -> ShoTermCmp/1("HwTq ")
  ActvCmpEna/2(LrngEnad) -> ShoTermCmp/5(LrngEnad)
  ShoTermCmp/1(ShoTermCmp) -> Calc_CmpTot/4(ShoTermCmp)
  If/1 -> If RstPer1 == True set RstPer1 to False/Action
  Data Store Read3/1 -> [SrvRst], If/1
  Calc_CmpTot/1(TotCmp) -> PullCmpCmd/1
  [PullCmpCmdDi] -> Calc_CmpTot/2(CmdDi)
  [VehSpd] -> Calc_CmpTot/1(VehSpd)
  [HwTq] -> FilLpUpdOutp/1
  RampDownStepSizeShoTerm/1 -> ShoTermCmp/3(RampDownStepSizeShoTerm)
  [SrvRst] -> Calc_CmpTot/3(SrvRst)
  VehLatA/1 -> ActvCmpEna/10(VehLatA)
  [PullCmpActvDi] -> Calc_CmpTot/5(PullCmpActvDi)
  PullCmpActvDi/1 -> [PullCmpActvDi]
  [PullCmpActvDi] -> Logical Operator/3
  ActvCmpEna/1(ShoTermRst) -> ShoTermCmp/4(ShoTermRst)

== system SF013A_PullCmpActv/PullCmpActv/PullCmpActvPer2/CopyRight2 ==

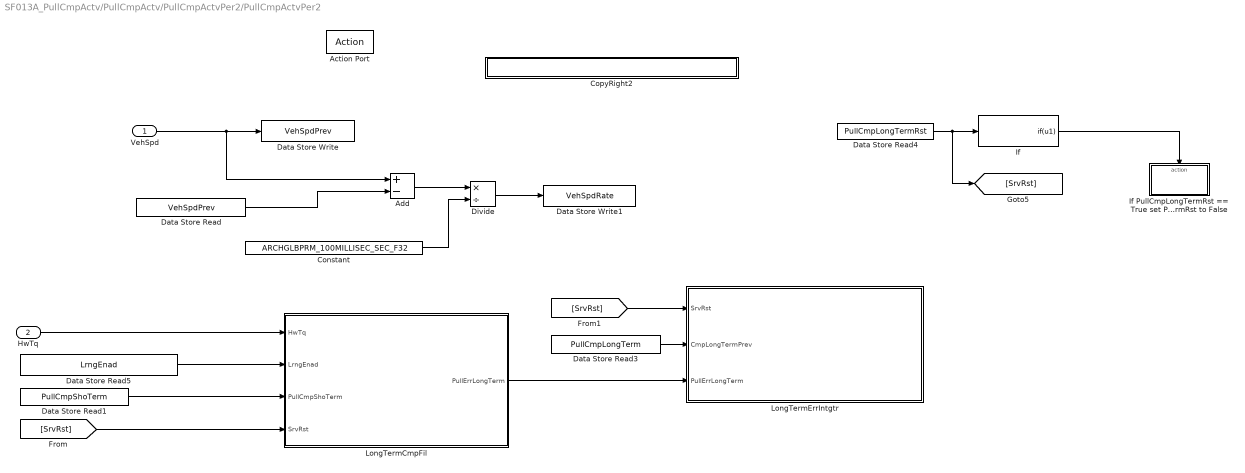
== system SF013A_PullCmpActv/PullCmpActv/PullCmpActvPer2/PullCmpActvPer2 ==
  VehSpd : Inport
  HwTq : Inport  Port=2
  Action Port : ActionPort  ActionType=then
  Add : Sum  Inputs=+-
  Constant : Constant  Value=ARCHGLBPRM_100MILLISEC_SEC_F32
  CopyRight2 : Subsystem  Description=|  mask(Copyright Information){none=on}
      | Copyright info block.                                               
      |                                                                     
      | Place copyright information at the top of every subsystem in design.
      mask prompts: none "No parameters"
      mask help: Place copyright information at the top of every subsystem in design.
      mask Display:
      | NxtrConf = 'Nexteer Confidential';
      | 
      | sys = bdroot; %handle for the current model ("system")
      | first = get_param(sys,'Created');
      | if(isempty(first))
      |     first = datestr(now,'yyyy');
      | else
      |     first = first(end-3:end);  %year is last four digits
      | end
      | 
      | last = get_param(sys,'LastModifiedDate');
      | if isempty(last)
      |     last = datestr(now,'yyyy');
      | else
      |     last = last(end-3:end);
      | end
      | 
      | if strcmp(first,last)
      |     fprintf('%s -- Copyright %s Nexteer',NxtrConf,first)
      | else
      |     fprintf('%s -- %s%s- %s Nexteer',NxtrConf,char(169),first,last)
      | end
  Data Store Read : DataStoreRead  Priority=1  DataStoreName=VehSpdPrev
      settings: AttributesFormatString=priority: %<Priority>
  Data Store Read1 : DataStoreRead  DataStoreName=PullCmpShoTerm
  Data Store Read3 : DataStoreRead  DataStoreName=PullCmpLongTerm
  Data Store Read4 : DataStoreRead  Priority=1  DataStoreName=PullCmpLongTermRst
      settings: AttributesFormatString=priority: %<Priority>
  Data Store Read5 : DataStoreRead  DataStoreName=LrngEnad
  Data Store Write : DataStoreWrite  Priority=2  DataStoreName=VehSpdPrev
      settings: AttributesFormatString=priority: %<Priority>
  Data Store Write1 : DataStoreWrite  DataStoreName=VehSpdRate
  Divide : Product  Inputs=*/
  If : If  IfExpression=u1  ShowElse=off
  If PullCmpLongTermRst == True set PullCmpLongTermRst to False : Subsystem  TreatAsAtomicUnit=on
  LongTermCmpFil : Subsystem  TreatAsAtomicUnit=on
  "LongTermErrIntgtr " : Subsystem  TreatAsAtomicUnit=on
  wires:
  VehSpd/1 -> Add/1, Data Store Write/1
  Data Store Read/1 -> Add/2
  Add/1 -> Divide/1
  Constant/1 -> Divide/2
  Divide/1 -> Data Store Write1/1
  HwTq/1 -> LongTermCmpFil/1("HwTq ")
  [SrvRst] -> LongTermCmpFil/4(SrvRst)
  Data Store Read5/1 -> LongTermCmpFil/2(LrngEnad)
  LongTermCmpFil/1(PullErrLongTerm) -> "LongTermErrIntgtr "/3(PullErrLongTerm)
  Data Store Read3/1 -> "LongTermErrIntgtr "/2(CmpLongTermPrev)
  If/1 -> If PullCmpLongTermRst == True set PullCmpLongTermRst to False/Action
  Data Store Read4/1 -> [SrvRst], If/1
  [SrvRst] -> "LongTermErrIntgtr "/1("SrvRst ")
  Data Store Read1/1 -> LongTermCmpFil/3(PullCmpShoTerm)

== system SF013A_PullCmpActv/PullCmpActv/RstPullCmp/CopyRight2 ==

== system SF013A_PullCmpActv/PullCmpActv/SetPullCmpLongTerm/CopyRight2 ==

== system SF013A_PullCmpActv/PullCmpActv/SetPullCmpShoTerm/CopyRight2 ==

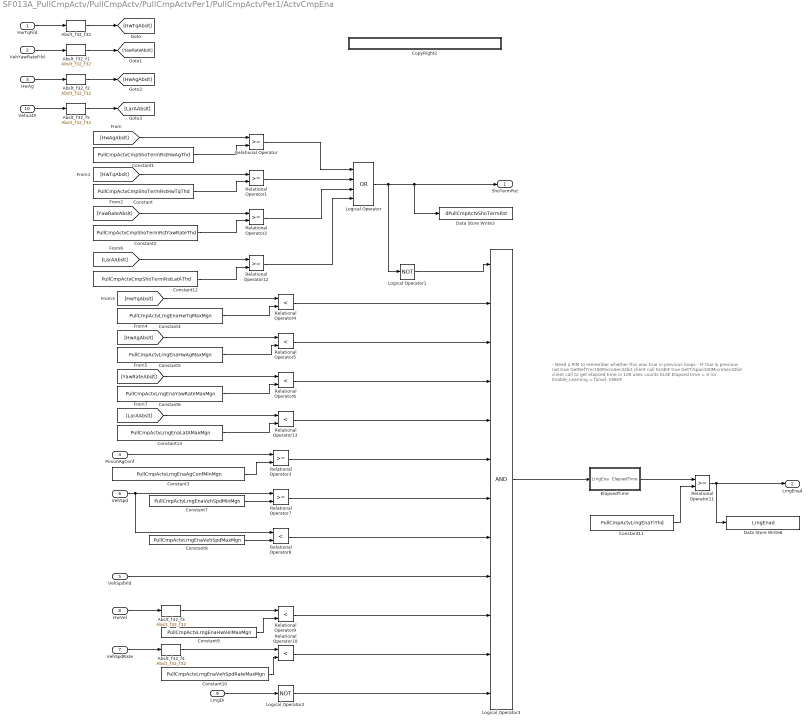
== system SF013A_PullCmpActv/PullCmpActv/PullCmpActvPer1/PullCmpActvPer1/ActvCmpEna ==
  note: -  Need a PIM to remember whether this was true in previous loops
      | -  IF true & previous not true
      |           GetRefTmr100MicroSec32bit client call
      |    ELSEIF  true
      |           GetTiSpan100MicroSec32bit client call to get elapsed time in 100 uSec counts
      |    ELSE
      |           Elapsed time = 0 (or Enable_Learning = false).
      |   ENDIF
  HwTqFild : Inport
  VehYawRateFild : Inport  Port=2
  HwAg : Inport  Port=3
  PinionAgConf : Inport  Port=4
  VehSpdVld : Inport  Port=5
  VehSpd : Inport  Port=6
  VehSpdRate : Inport  Port=7
  HwVel : Inport  Port=8
  LrngDi : Inport  Port=9
  VehLatA : Inport  Port=10
  Abslt_f32_f{1..5,32} (6 alike) : NxtrAbslt/Abslt_f32_f32  SFunctionSpec=single y1 = Abslt_f32_f32(single u1)
      settings: AttributesFormatString=%<Name>
  Constant : Constant  Value=PullCmpActvCmpShoTermRstHwTqThd
  Constant1 : Constant  Value=PullCmpActvCmpShoTermRstHwAgThd
  Constant10 : Constant  Value=PullCmpActvLrngEnaVehSpdRateMaxMgn
  Constant11 : Constant  Value=PullCmpActvLrngEnaTiThd
  Constant12 : Constant  Value=PullCmpActvCmpShoTermRstLatAThd
  Constant13 : Constant  Value=PullCmpActvLrngEnaLatAMaxMgn
  Constant2 : Constant  Value=PullCmpActvCmpShoTermRstYawRateThd
  Constant3 : Constant  Value=PullCmpActvLrngEnaAgConfMinMgn
  Constant4 : Constant  Value=PullCmpActvLrngEnaHwTqMaxMgn
  Constant5 : Constant  Value=PullCmpActvLrngEnaHwAgMaxMgn
  Constant6 : Constant  Value=PullCmpActvLrngEnaYawRateMaxMgn
  Constant7 : Constant  Value=PullCmpActvLrngEnaVehSpdMinMgn
  Constant8 : Constant  Value=PullCmpActvLrngEnaVehSpdMaxMgn
  Constant9 : Constant  Value=PullCmpActvLrngEnaHwVelMaxMgn
  CopyRight2 : Subsystem  Description=|  mask(Copyright Information){none=on}
      | Copyright info block.                                               
      |                                                                     
      | Place copyright information at the top of every subsystem in design.
      mask prompts: none "No parameters"
      mask help: Place copyright information at the top of every subsystem in design.
      mask Display:
      | NxtrConf = 'Nexteer Confidential';
      | 
      | sys = bdroot; %handle for the current model ("system")
      | first = get_param(sys,'Created');
      | if(isempty(first))
      |     first = datestr(now,'yyyy');
      | else
      |     first = first(end-3:end);  %year is last four digits
      | end
      | 
      | last = get_param(sys,'LastModifiedDate');
      | if isempty(last)
      |     last = datestr(now,'yyyy');
      | else
      |     last = last(end-3:end);
      | end
      | 
      | if strcmp(first,last)
      |     fprintf('%s -- Copyright %s Nexteer',NxtrConf,first)
      | else
      |     fprintf('%s -- %s%s- %s Nexteer',NxtrConf,char(169),first,last)
      | end
  Data Store Write3 : DataStoreWrite  DataStoreName=dPullCmpActvShoTermRst
  Data Store Write6 : DataStoreWrite  DataStoreName=LrngEnad
  ElapsedTime : Subsystem  TreatAsAtomicUnit=on
  Logical Operator : Logic  Operator=OR  Inputs=4  AllPortsSameDT=off  OutDataTypeStr=boolean
  Logical Operator1 : Logic  Operator=NOT  Inputs=1  AllPortsSameDT=off  OutDataTypeStr=boolean
  Logical Operator2 : Logic  Operator=NOT  Inputs=1  AllPortsSameDT=off  OutDataTypeStr=boolean
  Logical Operator3 : Logic  Inputs=12  AllPortsSameDT=off  OutDataTypeStr=boolean
  Relational Operator{,1..3,7,11..12} (7 alike) : RelationalOperator  OutDataTypeStr=boolean
  Relational Operator{4..6,8..10,13} (7 alike) : RelationalOperator  Operator=<  OutDataTypeStr=boolean
  ShoTermRst : Outport
  LrngEnad : Outport  Port=2
  wires:
  HwTqFild/1 -> Abslt_f32_f32/1
  VehYawRateFild/1 -> Abslt_f32_f1/1
  HwAg/1 -> Abslt_f32_f2/1
  Abslt_f32_f2/1 -> [HwAgAbslt]
  Abslt_f32_f1/1 -> [YawRateAbslt]
  Abslt_f32_f32/1 -> [HwTqAbslt]
  [HwAgAbslt] -> Relational Operator/1
  [HwTqAbslt] -> Relational Operator1/1
  [YawRateAbslt] -> Relational Operator2/1
  Constant1/1 -> Relational Operator/2
  Constant/1 -> Relational Operator1/2
  Constant2/1 -> Relational Operator2/2
  Relational Operator/1 -> Logical Operator/1
  Relational Operator1/1 -> Logical Operator/2
  Relational Operator2/1 -> Logical Operator/3
  Logical Operator/1 -> Logical Operator1/1, Data Store Write3/1, ShoTermRst/1
  PinionAgConf/1 -> Relational Operator3/1
  Constant3/1 -> Relational Operator3/2
  [HwTqAbslt] -> Relational Operator4/1
  Constant4/1 -> Relational Operator4/2
  [HwAgAbslt] -> Relational Operator5/1
  Constant5/1 -> Relational Operator5/2
  [YawRateAbslt] -> Relational Operator6/1
  Constant6/1 -> Relational Operator6/2
  VehSpd/1 -> Relational Operator8/1, Relational Operator7/1
  Constant7/1 -> Relational Operator7/2
  Constant8/1 -> Relational Operator8/2
  HwVel/1 -> Abslt_f32_f3/1
  Constant9/1 -> Relational Operator9/2
  Abslt_f32_f3/1 -> Relational Operator9/1
  VehSpdRate/1 -> Abslt_f32_f4/1
  Abslt_f32_f4/1 -> Relational Operator10/1
  Constant10/1 -> Relational Operator10/2
  LrngDi/1 -> Logical Operator2/1
  Relational Operator4/1 -> Logical Operator3/2
  Relational Operator5/1 -> Logical Operator3/3
  Relational Operator6/1 -> Logical Operator3/4
  Logical Operator1/1 -> Logical Operator3/1
  Logical Operator3/1 -> ElapsedTime/1(LrngEna)
  ElapsedTime/1(ElapsedTime) -> Relational Operator11/1
  Constant11/1 -> Relational Operator11/2
  Relational Operator11/1 -> Data Store Write6/1, LrngEnad/1
  VehLatA/1 -> Abslt_f32_f5/1
  Abslt_f32_f5/1 -> [LarAAbslt]
  [LarAAbslt] -> Relational Operator12/1
  Constant12/1 -> Relational Operator12/2
  Relational Operator12/1 -> Logical Operator/4
  Constant13/1 -> Relational Operator13/2
  Relational Operator13/1 -> Logical Operator3/5
  [LarAAbslt] -> Relational Operator13/1
  Relational Operator3/1 -> Logical Operator3/6
  Relational Operator7/1 -> Logical Operator3/7
  Relational Operator8/1 -> Logical Operator3/8
  VehSpdVld/1 -> Logical Operator3/9
  Relational Operator9/1 -> Logical Operator3/10
  Relational Operator10/1 -> Logical Operator3/11
  Logical Operator2/1 -> Logical Operator3/12
